simulink model "RC_circut"  (R2023b)
settings: Solver=VariableStepAuto  StartTime=0.0  StopTime=10.0
values from neighbouring files (symbols this model uses):
  C = 1e-6    (= 1e-06)    [RC_circut_parameters.m]    (also in trial_pend.m)
  R = 1e3    (= 1000)    [RC_circut_parameters.m]    (also in trial_pend.m = 5)
settings Model: VariantFading=off  Creator=DELL  LastModifiedBy=DELL

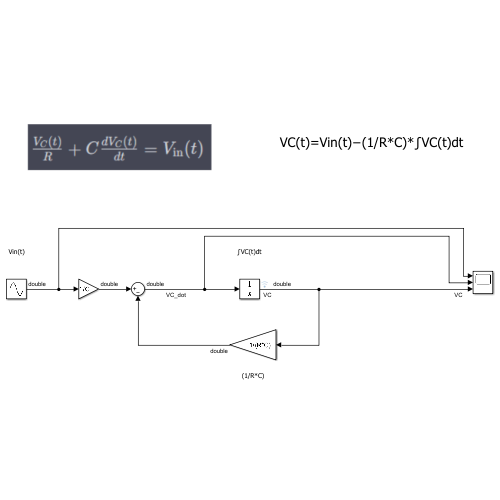
[thumbnail: Simulink's stored preview of the top-level diagram]
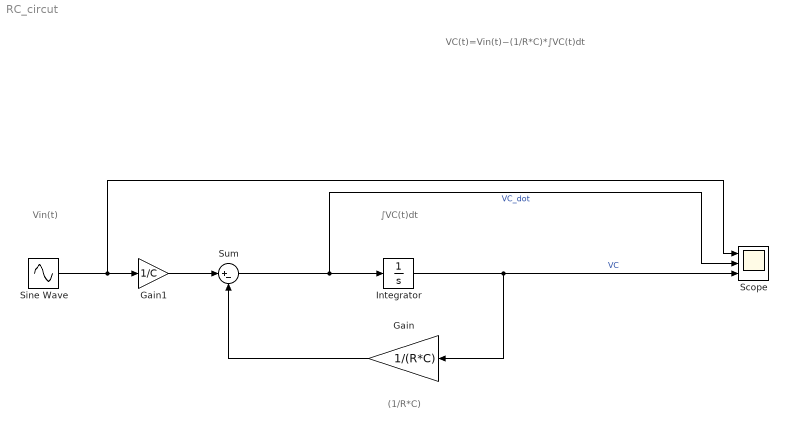
== system RC_circut ==
  note: ​∫VC​(t)dt
  note: (1/R*C)
  note: Vin​(t)
  note: VC​(t)=Vin​(t)−(1/R*C)*​∫VC​(t)dt
  Gain : Gain  Gain=1/(R*C)
  Gain1 : Gain  Gain=1/C
  Integrator : Integrator  InitialCondition=1
  Scope : Scope  NumInputPorts=3
  Sine Wave : Sin  Amplitude=5  Frequency=2*pi  SampleTime=0
  Sum : Sum  Inputs=|+-
  wires:
  Sum/1 -> Scope/2, Integrator/1  "VC_dot"
  Integrator/1 -> Gain/1, Scope/3  "VC"
  Gain/1 -> Sum/2
  Sine Wave/1 -> Scope/1, Gain1/1
  Gain1/1 -> Sum/1
